simulink model "Additional_Import"  (Simulink 7.0)
settings: Solver=ode45  StartTime=0.0  StopTime=10.0  RelTol=1e-3
libraries: simulink x1
settings Model: Creator=Administrator  LastModifiedBy=Nag

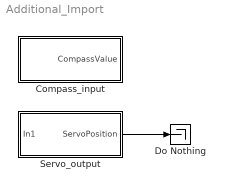
== system Additional_Import ==
  Compass_input : Subsystem
  Do Nothing : Terminator
  Servo_output : Subsystem
  wires:
  Servo_output/1(ServoPosition) -> Do Nothing/1

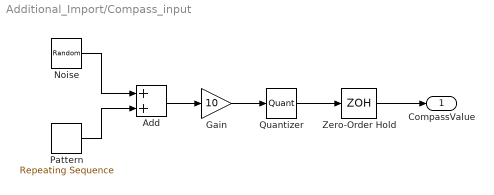
== system Additional_Import/Compass_input ==
  Add : Sum  OutDataType=sfix(16)  OutScaling=2^-10
  Gain : Gain  Gain=10  ParameterDataType=sfix(16)  ParameterScaling=2^0  OutDataType=sfix(16)  OutScaling=2^0
  Noise : RandomNumber  SampleTime=0
  Pattern : simulink/Sources/Repeating Sequence  SystemSampleTime=-1  rep_seq_t=[0 10]  rep_seq_y=[0 360]
  Quantizer : Quantizer  QuantizationInterval=1
  Zero-Order Hold : ZeroOrderHold  SampleTime=1/8
  CompassValue : Outport  OutDataType=sfix(16)  OutScaling=2^0
  wires:
  Noise/1 -> Add/1
  Pattern/1 -> Add/2
  Zero-Order Hold/1 -> CompassValue/1
  Add/1 -> Gain/1
  Gain/1 -> Quantizer/1
  Quantizer/1 -> Zero-Order Hold/1

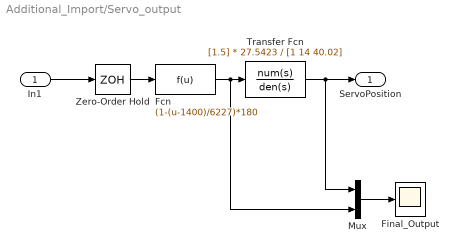
== system Additional_Import/Servo_output ==
  In1 : Inport  OutDataType=sfix(16)  OutScaling=2^0
  Fcn : Fcn  Expr=(1-(u-1400)/6227)*180  SampleTime=1/8
  Final_Output : Scope
      settings: YMin=20  YMax=180  SaveName=ScopeData6
  Mux : Mux  Inputs=2
  Transfer Fcn : TransferFcn  Numerator=[1.5] * 27.5423  Denominator=[1 14 40.02]
  Zero-Order Hold : ZeroOrderHold  SampleTime=1/8
  ServoPosition : Outport  OutDataType=sfix(16)  OutScaling=2^0
  wires:
  Transfer Fcn/1 -> ServoPosition/1, Mux/1
  In1/1 -> Zero-Order Hold/1
  Fcn/1 -> Mux/2, Transfer Fcn/1
  Zero-Order Hold/1 -> Fcn/1
  Mux/1 -> Final_Output/1
